simulink model "test2"  (R2017b)
settings: Solver=VariableStepAuto  StartTime=0.0  StopTime=100.0  RelTol=1e-3
settings Model: Creator=mountaintop  LastModifiedBy=mountaintop

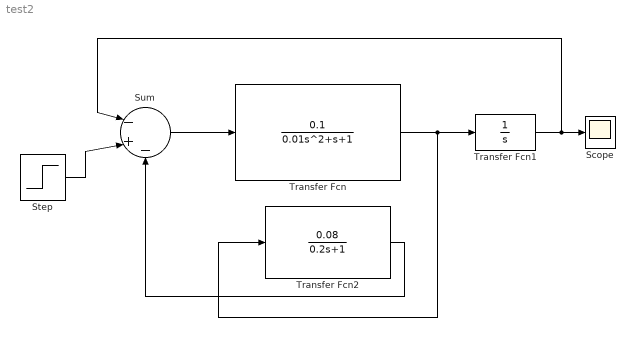
== system test2 ==
  Scope : Scope
  Step : Step  SampleTime=0
  Sum : Sum  Inputs=|-+-
  Transfer Fcn : TransferFcn  Numerator=[0.1]  Denominator=[0.01 1 1]
  Transfer Fcn1 : TransferFcn  Denominator=[1 0]
  Transfer Fcn2 : TransferFcn  Numerator=[0.08]  Denominator=[0.2 1]
  wires:
  Transfer Fcn1/1 -> Sum/1, Scope/1
  Transfer Fcn/1 -> Transfer Fcn2/1, Transfer Fcn1/1
  Transfer Fcn2/1 -> Sum/3
  Sum/1 -> Transfer Fcn/1
  Step/1 -> Sum/2
